simulink model "LAHernandez22210415"  (R2023a)
settings: Solver=ode15s  StartTime=0.0  StopTime=10.0  MaxStep=1e-3  RelTol=1e-3
settings Model: Creator=piqui  LastModifiedBy=piqui
settings DataIOCC: ReturnWorkspaceOutputs=off  TimeSaveName=t
settings DebuggingCC: AlgebraicLoopMsg=none  ArtificialAlgebraicLoopMsg=none  BlockPriorityViolationMsg=error  MinStepSizeMsg=error  MaxConsecutiveZCsMsg=none  ModelReferenceExtraNoncontSigs=none  OperatingPointInterfaceChecksumMismatchMsg=error

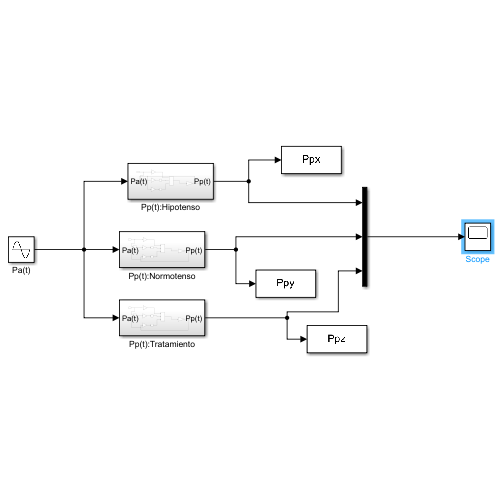
[thumbnail: Simulink's stored preview of the top-level diagram]
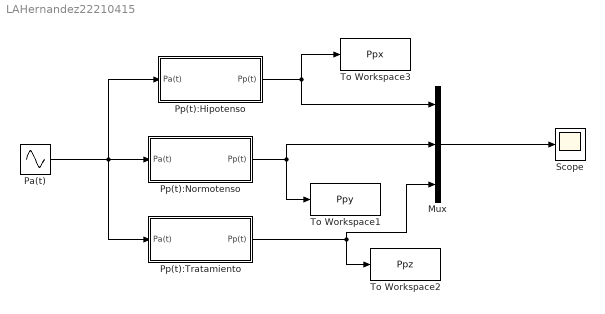
== system LAHernandez22210415 ==
  Mux : Mux  Inputs=3
  Pa(t) : Sin  Amplitude=2.5  Frequency=(2*pi)  SampleTime=0
  Pp(t):Hipotenso : Subsystem
  Pp(t):Normotenso : Subsystem
  Pp(t):Tratamiento : Subsystem
  Scope : Scope
  To Workspace1 : ToWorkspace  VariableName=Ppy  SampleTime=-1
  To Workspace2 : ToWorkspace  VariableName=Ppz  SampleTime=-1
  To Workspace3 : ToWorkspace  VariableName=Ppx  SampleTime=-1
  wires:
  Mux/1 -> Scope/1
  Pa(t)/1 -> Pp(t):Tratamiento/1(Pa(t)), Pp(t):Hipotenso/1(Pa(t)), Pp(t):Normotenso/1(Pa(t))
  Pp(t):Hipotenso/1(Pp(t)) -> Mux/1, To Workspace3/1
  Pp(t):Normotenso/1(Pp(t)) -> Mux/2, To Workspace1/1
  Pp(t):Tratamiento/1(Pp(t)) -> Mux/3, To Workspace2/1

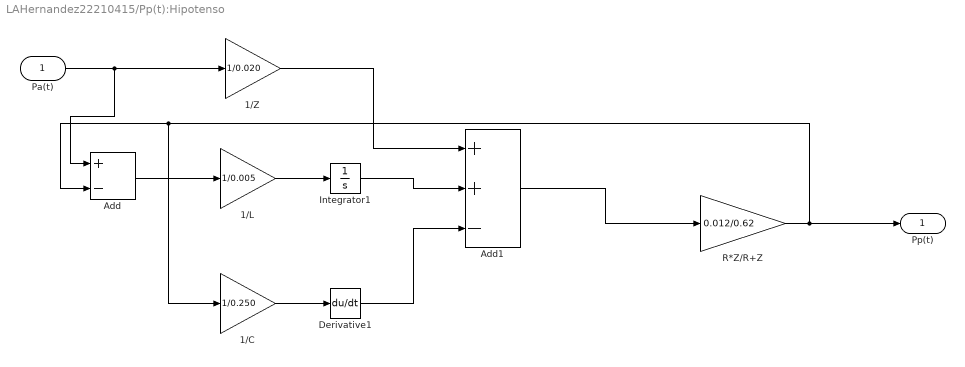
== system LAHernandez22210415/Pp(t):Hipotenso ==
  Pa(t) : Inport
  1/C : Gain  Gain=1/0.250
  1/L : Gain  Gain=1/0.005
  1/Z : Gain  Gain=1/0.020
  Add : Sum  Inputs=+-
  Add1 : Sum  Inputs=++-
  Derivative1 : Derivative
  Integrator1 : Integrator
  R*Z/R+Z : Gain  Gain=0.012/0.62
  Pp(t) : Outport
  wires:
  1/L/1 -> Integrator1/1
  1/C/1 -> Derivative1/1
  Pa(t)/1 -> Add/1, 1/Z/1
  Add/1 -> 1/L/1
  Add1/1 -> R*Z/R+Z/1
  1/Z/1 -> Add1/1
  Integrator1/1 -> Add1/2
  Derivative1/1 -> Add1/3
  R*Z/R+Z/1 -> 1/C/1, Add/2, Pp(t)/1

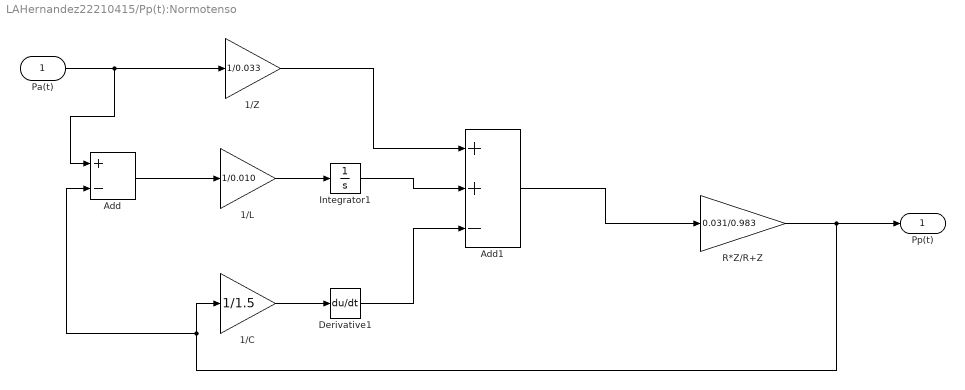
== system LAHernandez22210415/Pp(t):Normotenso ==
  Pa(t) : Inport
  1/C : Gain  Gain=1/1.5
  1/L : Gain  Gain=1/0.010
  1/Z : Gain  Gain=1/0.033
  Add : Sum  Inputs=+-
  Add1 : Sum  Inputs=++-
  Derivative1 : Derivative
  Integrator1 : Integrator
  R*Z/R+Z : Gain  Gain=0.031/0.983
  Pp(t) : Outport
  wires:
  1/L/1 -> Integrator1/1
  1/C/1 -> Derivative1/1
  Pa(t)/1 -> Add/1, 1/Z/1
  Add/1 -> 1/L/1
  Add1/1 -> R*Z/R+Z/1
  1/Z/1 -> Add1/1
  Integrator1/1 -> Add1/2
  Derivative1/1 -> Add1/3
  R*Z/R+Z/1 -> Add/2, 1/C/1, Pp(t)/1

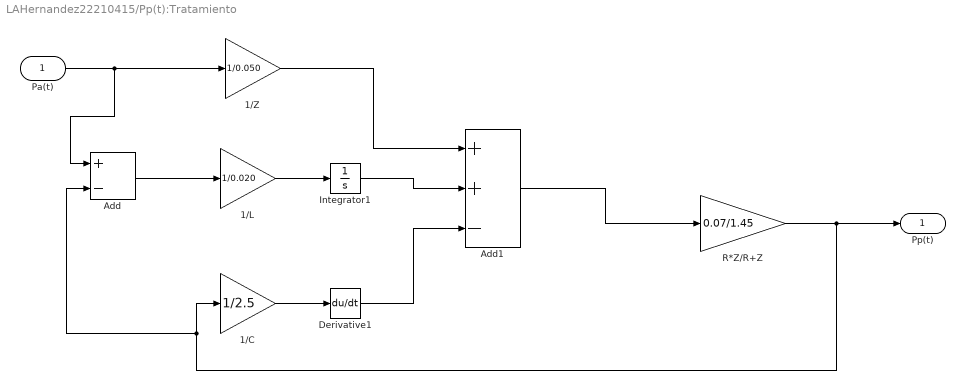
== system LAHernandez22210415/Pp(t):Tratamiento ==
  Pa(t) : Inport
  1/C : Gain  Gain=1/2.5
  1/L : Gain  Gain=1/0.020
  1/Z : Gain  Gain=1/0.050
  Add : Sum  Inputs=+-
  Add1 : Sum  Inputs=++-
  Derivative1 : Derivative
  Integrator1 : Integrator
  R*Z/R+Z : Gain  Gain=0.07/1.45
  Pp(t) : Outport
  wires:
  1/L/1 -> Integrator1/1
  1/C/1 -> Derivative1/1
  Pa(t)/1 -> Add/1, 1/Z/1
  Add/1 -> 1/L/1
  Add1/1 -> R*Z/R+Z/1
  1/Z/1 -> Add1/1
  Integrator1/1 -> Add1/2
  Derivative1/1 -> Add1/3
  R*Z/R+Z/1 -> Add/2, 1/C/1, Pp(t)/1
